simulink model "sampleModel1560"  (R2023a)
settings: Solver=VariableStepAuto  StartTime=0.0  StopTime=10.0  RelTol=1e-3
libraries: hdlsllib x2, simulink x2
settings Model: Creator=user1  LastModifiedBy=user1

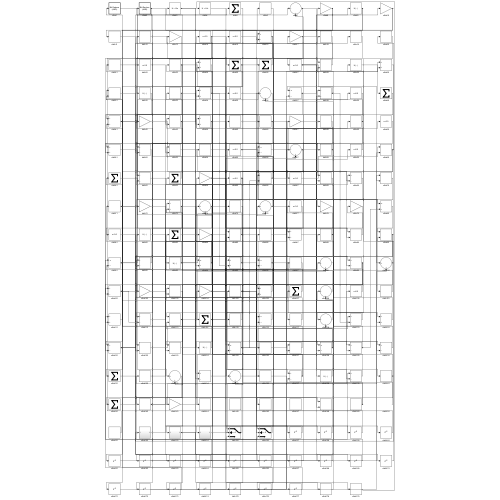
[thumbnail: Simulink's stored preview of the top-level diagram]
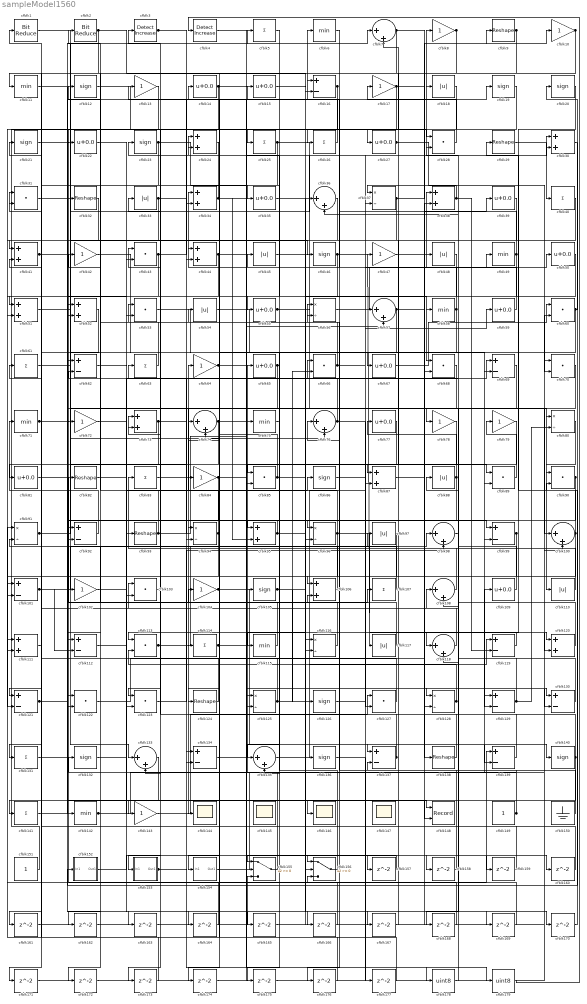
== system sampleModel1560 ==
  cfblk1 : hdlsllib/Logic and Bit Operations/Bit Reduce  mode=AND
  cfblk{8,10,13,17,42,47,64,72,78..79,84,102,104,143} (14 alike) : Gain
  cfblk{7,36,57,74,76,98,100,108,118,133,135} (11 alike) : Sum  Inputs=|++
  cfblk{16,62,69,92,99,101,112,119,121,129..130,134,137,139} (14 alike) : Sum  Inputs=+-
  cfblk{28,31,43,53,60,66,68,70,85,89..90,103,113,122..123,127} (16 alike) : DotProduct  OutDataTypeStr=Inherit: Inherit via internal rule
  cfblk{12,19..21,23,46,86,105,126,132,136,140} (12 alike) : Signum
  cfblk{24,30,34,38,41,44,51..52,73,87,95,106,111,120} (14 alike) : Sum
  cfblk{5,25..26,40,61,63,83,107,114,131,141} (11 alike) : Sum  Inputs=+
  cfblk{14..15,22,27,35,39,50,55,59,65,67,77,81,109} (14 alike) : Bias  Bias=0.0  SaturateOnIntegerOverflow=off
  cfblk{6,11,49,58,71,75,115,142} (8 alike) : MinMax
  cfblk{18,33,45,48,54,88,97,110,117} (9 alike) : Abs  SaturateOnIntegerOverflow=off
  cfblk{37,56,80,91,94,96,116,125,128} (9 alike) : Product  Inputs=*/  RndMeth=Zero  SaturateOnIntegerOverflow=on
  cfblk{9,29,32,82,93,124,138} (7 alike) : Reshape
  cfblk{144..147} (4 alike) : Scope
      cfblk145 settings: Floating=on
      cfblk147 settings: Floating=on
  cfblk148 : Record  FileSettingsInternal="{\"entries\":[{\"content\":{\"excelSettings\":{\"content\":{},\"type\":\"Streamout.ExcelSettings\"}},\"type\":\"Streamout.FileSettingStorage\",\"uuid\":\"\"}],\"packageUris\":[\"http:\\/\\/schema.mathworks.com\\/mf0\\/streamout_blocks\\/R2020a\"],\"version\":\"1.0\"}"  Layout=[1 1]  SignalsInternal="{\"entries\":[{\"content\":{\"signals\":[{\"content\":{\"blockPath\":[],\"dimensions\":[1],\"domain\":\"\",\"lineColor\":\"#a2142f\",\"plots\":[1],\"port\":1,\"signalID\":1701,\"signalName\":\"XY Graph:1\"},\"type\":\"RecordBlkView.Signal\",\"uuid\":\"\"},{\"content\":{\"blockPath\":[],\"dimensions\":[1],\"domain\":\"\",\"lineColor\":\"#139fff\",\"plots\":[1],\"port\":2,\"signalID\":1704,\"signalName\":\"XY Graph:2\"},\"type\":\"RecordBlkView.Signal\",\"uuid\":\"\"}]},\"type\":\"RecordBlkView.InputSignals\",\"uuid\":\"\"}],\"packageUris\":[\"http:\\/\\/schema.mathworks.com\\/mf0\\/streamout_blocks\\/R2020a\"],\"version\":\"1.0\"}"  VisualizationBindings="{\"xyplotplugin\":{\"info\":[{\"series\":[{\"bindingParametersList\":[{\"parameter\":\"X-Axis\",\"signalID\":1701,\"signalName\":\"XY Graph:1\"},{\"parameter\":\"Y-Axis\",\"signalID\":1704,\"signalName\":\"XY Graph:2\"}],\"seriesID\":51913}],\"subplotID\":1}]}}"  CompatibilityTag=XY  st=-1
  cfblk149 : Constant  SampleTime=-1
  cfblk150 : Ground
  cfblk151 : Constant  SampleTime=-1
  cfblk152 : Subsystem
      settings: LibrarySourceBlock=|
      | hdlsllib/Ports &
      | Subsystems/Subsystem
  cfblk153 : Subsystem
      settings: LibrarySourceBlock=|
      | hdlsllib/Ports &
      | Subsystems/Subsystem
  cfblk154 : Subsystem
      settings: LibrarySourceBlock=|
      | hdlsllib/Ports &
      | Subsystems/Subsystem
  cfblk155 : Switch  SaturateOnIntegerOverflow=off  InputSameDT=off
  cfblk156 : Switch  SaturateOnIntegerOverflow=off  InputSameDT=off
  cfblk{157..177} (21 alike) : Delay  SampleTime=1
  cfblk178 : DataTypeConversion  OutDataTypeStr=uint8  SaturateOnIntegerOverflow=off  RndMeth=Floor
  cfblk179 : DataTypeConversion  OutDataTypeStr=uint8  SaturateOnIntegerOverflow=off  RndMeth=Floor
  cfblk2 : hdlsllib/Logic and Bit Operations/Bit Reduce  mode=AND
  cfblk3 : simulink/Logic and Bit Operations/Detect Increase  vinit=0.0  OutDataTypeStr=boolean
      settings: LibrarySourceBlock=|
      | hdlsllib/Logic and Bit
      | Operations/Detect
      | Increase
  cfblk4 : simulink/Logic and Bit Operations/Detect Increase  vinit=0.0  OutDataTypeStr=boolean
      settings: LibrarySourceBlock=|
      | hdlsllib/Logic and Bit
      | Operations/Detect
      | Increase
  wires:
  cfblk109/1 -> cfblk63/1
  cfblk143/1 -> cfblk127/1
  cfblk108/1 -> cfblk83/1
  cfblk20/1 -> cfblk118/1
  cfblk55/1 -> cfblk110/1, cfblk58/1
  cfblk98/1 -> cfblk118/2
  cfblk119/1 -> cfblk113/1
  cfblk28/1 -> cfblk17/1
  cfblk82/1 -> cfblk93/1
  cfblk36/1 -> cfblk133/1
  cfblk89/1 -> cfblk79/1
  cfblk21/1 -> cfblk139/1
  cfblk132/1 -> cfblk86/1
  cfblk104/1 -> cfblk137/1, cfblk97/1
  cfblk130/1 -> cfblk45/1
  cfblk151/1 -> cfblk25/1
  cfblk46/1 -> cfblk117/1, cfblk51/2
  cfblk101/1 -> cfblk98/1, cfblk112/2
  cfblk25/1 -> cfblk78/1, cfblk43/2
  cfblk92/1 -> cfblk71/1
  cfblk80/1 -> cfblk90/1
  cfblk45/1 -> cfblk80/1
  cfblk67/1 -> cfblk60/1
  cfblk91/1 -> cfblk7/1, cfblk99/2
  cfblk88/1 -> cfblk77/1, cfblk156/1
  cfblk30/1 -> cfblk152/1(In1)
  cfblk26/1 -> cfblk6/1
  cfblk127/1 -> cfblk31/1
  cfblk57/1 -> cfblk89/2, cfblk174/1
  cfblk103/1 -> cfblk153/1(In1)
  cfblk115/1 -> cfblk82/1
  cfblk1/1 -> cfblk76/2
  cfblk29/1 -> cfblk40/1
  cfblk42/1 -> cfblk129/1
  cfblk138/1 -> cfblk65/1
  cfblk68/1 -> cfblk144/1
  cfblk74/1 -> cfblk131/1, cfblk19/1
  cfblk83/1 -> cfblk64/1
  cfblk155/1 -> cfblk105/1
  cfblk77/1 -> cfblk135/1
  cfblk110/1 -> cfblk73/1
  cfblk59/1 -> cfblk34/1
  cfblk44/1 -> cfblk139/2, cfblk52/1
  cfblk52/1 -> cfblk81/1
  cfblk100/1 -> cfblk29/1, cfblk114/1
  cfblk135/1 -> cfblk47/1
  cfblk93/1 -> cfblk75/1, cfblk42/1, cfblk66/1
  cfblk8/1 -> cfblk124/1, cfblk55/1
  cfblk154/1(Out1) -> cfblk109/1
  cfblk153/1(Out1) -> cfblk156/3, cfblk179/1
  cfblk2/1 -> cfblk11/1, cfblk16/2
  cfblk9/1 -> cfblk27/1, cfblk171/1
  cfblk137/1 -> cfblk14/1, cfblk24/2
  cfblk96/1 -> cfblk138/1, cfblk134/2, cfblk3/1
  cfblk128/1 -> cfblk56/1, cfblk113/2
  cfblk43/1 -> cfblk142/1, cfblk18/1
  cfblk125/1 -> cfblk44/1, cfblk119/1, cfblk66/2
  cfblk124/1 -> cfblk61/1
  cfblk140/1 -> cfblk141/1, cfblk73/2
  cfblk141/1 -> cfblk15/1
  cfblk112/1 -> cfblk69/1
  cfblk95/1 -> cfblk94/1, cfblk128/1
  cfblk149/1 -> cfblk132/1, cfblk137/2
  cfblk40/1 -> cfblk154/1(In1)
  cfblk47/1 -> cfblk38/1
  cfblk113/1 -> cfblk50/1, cfblk133/2
  cfblk56/1 -> cfblk48/1
  cfblk122/1 -> cfblk39/1
  cfblk33/1 -> cfblk121/1, cfblk165/1
  cfblk94/1 -> cfblk53/1, cfblk2/1, cfblk123/2
  cfblk156/1 -> cfblk23/1
  cfblk97/1 -> cfblk115/1
  cfblk71/1 -> cfblk134/1, cfblk148/1
  cfblk35/1 -> cfblk68/1
  cfblk34/1 -> cfblk32/1, cfblk87/2, cfblk95/2
  cfblk10/1 -> cfblk106/1, cfblk112/1
  cfblk19/1 -> cfblk96/1
  cfblk3/1 -> cfblk26/1, cfblk148/2
  cfblk106/1 -> cfblk24/1
  cfblk41/1 -> cfblk8/1, cfblk46/1
  cfblk66/1 -> cfblk33/1, cfblk49/1
  cfblk139/1 -> cfblk56/2
  cfblk13/1 -> cfblk101/2
  cfblk48/1 -> cfblk87/1
  cfblk63/1 -> cfblk12/1
  cfblk105/1 -> cfblk126/1, cfblk130/2, cfblk157/1
  cfblk16/1 -> cfblk22/1, cfblk173/1
  cfblk39/1 -> cfblk67/1
  cfblk31/1 -> cfblk53/2
  cfblk53/1 -> cfblk68/2
  cfblk90/1 -> cfblk108/2, cfblk122/2
  cfblk129/1 -> cfblk103/1, cfblk80/2
  cfblk12/1 -> cfblk155/2
  cfblk58/1 -> cfblk96/2, cfblk16/1
  cfblk65/1 -> cfblk72/1, cfblk95/1
  cfblk51/1 -> cfblk69/2
  cfblk14/1 -> cfblk44/2, cfblk89/1, cfblk52/2
  cfblk107/1 -> cfblk31/2
  cfblk123/1 -> cfblk98/2
  cfblk7/1 -> cfblk41/1, cfblk130/1
  cfblk76/1 -> cfblk129/2, cfblk43/1
  cfblk84/1 -> cfblk122/1, cfblk127/2
  cfblk22/1 -> cfblk99/1
  cfblk17/1 -> cfblk146/1, cfblk9/1
  cfblk38/1 -> cfblk37/1, cfblk119/2
  cfblk121/1 -> cfblk5/1, cfblk107/1, cfblk164/1
  cfblk142/1 -> cfblk70/1, cfblk104/1
  cfblk11/1 -> cfblk28/1
  cfblk87/1 -> cfblk120/1
  cfblk111/1 -> cfblk91/2
  cfblk126/1 -> cfblk30/1
  cfblk5/1 -> cfblk35/1
  cfblk23/1 -> cfblk125/1, cfblk51/1, cfblk143/1
  cfblk116/1 -> cfblk84/1
  cfblk27/1 -> cfblk70/2, cfblk120/2, cfblk140/1
  cfblk99/1 -> cfblk121/2, cfblk123/1, cfblk172/1
  cfblk49/1 -> cfblk13/1, cfblk92/2
  cfblk64/1 -> cfblk116/2, cfblk159/1
  cfblk61/1 -> cfblk100/1
  cfblk78/1 -> cfblk103/2
  cfblk73/1 -> cfblk102/1, cfblk170/1
  cfblk117/1 -> cfblk92/1
  cfblk134/1 -> cfblk57/2
  cfblk60/1 -> cfblk85/1, cfblk20/1, cfblk156/2
  cfblk75/1 -> cfblk135/2
  cfblk102/1 -> cfblk85/2
  cfblk32/1 -> cfblk62/1
  cfblk54/1 -> cfblk136/1
  cfblk69/1 -> cfblk74/2
  cfblk150/1 -> cfblk28/2
  cfblk18/1 -> cfblk94/2
  cfblk37/1 -> cfblk111/2, cfblk10/1
  cfblk86/1 -> cfblk59/1
  cfblk85/1 -> cfblk62/2, cfblk128/2
  cfblk120/1 -> cfblk36/2
  cfblk24/1 -> cfblk34/2
  cfblk118/1 -> cfblk21/1
  cfblk114/1 -> cfblk106/2, cfblk30/2
  cfblk157/1 -> cfblk155/1
  cfblk152/1(Out1) -> cfblk158/1
  cfblk158/1 -> cfblk76/1
  cfblk159/1 -> cfblk1/1
  cfblk62/1 -> cfblk160/1
  cfblk160/1 -> cfblk116/1
  cfblk133/1 -> cfblk161/1
  cfblk161/1 -> cfblk36/1
  cfblk50/1 -> cfblk162/1
  cfblk162/1 -> cfblk155/3
  cfblk81/1 -> cfblk163/1
  cfblk163/1 -> cfblk38/2
  cfblk164/1 -> cfblk91/1
  cfblk165/1 -> cfblk100/2
  cfblk131/1 -> cfblk166/1
  cfblk166/1 -> cfblk101/1
  cfblk72/1 -> cfblk167/1
  cfblk167/1 -> cfblk7/2
  cfblk70/1 -> cfblk168/1
  cfblk168/1 -> cfblk74/1
  cfblk15/1 -> cfblk169/1
  cfblk169/1 -> cfblk108/1
  cfblk170/1 -> cfblk90/2
  cfblk171/1 -> cfblk125/2
  cfblk172/1 -> cfblk37/2
  cfblk173/1 -> cfblk41/2
  cfblk174/1 -> cfblk60/2
  cfblk79/1 -> cfblk175/1
  cfblk175/1 -> cfblk57/1
  cfblk6/1 -> cfblk176/1
  cfblk176/1 -> cfblk111/1
  cfblk136/1 -> cfblk177/1
  cfblk177/1 -> cfblk54/1
  cfblk4/1 -> cfblk178/1
  cfblk178/1 -> cfblk88/1
  cfblk179/1 -> cfblk4/1

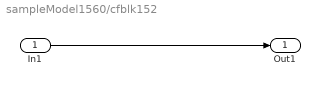
== system sampleModel1560/cfblk152 ==
  In1 : Inport
  Out1 : Outport
  wires:
  In1/1 -> Out1/1

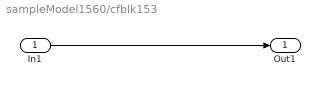
== system sampleModel1560/cfblk153 ==
  In1 : Inport
  Out1 : Outport
  wires:
  In1/1 -> Out1/1

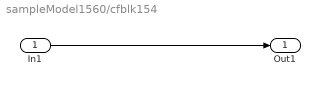
== system sampleModel1560/cfblk154 ==
  In1 : Inport
  Out1 : Outport
  wires:
  In1/1 -> Out1/1
